simulink model "DynamicCenterGravity_TestModel"  (R2014a)
settings: Solver=ode45  StartTime=0.0  StopTime=10.0  RelTol=1e-3
libraries: rocket_dynamic_data_library x1
settings Model: Creator=scorpii  LastModifiedBy=scorpii

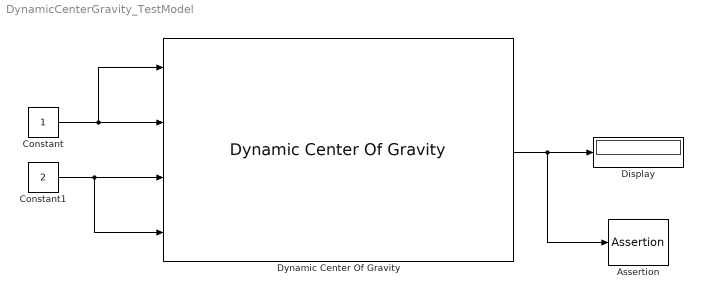
== system DynamicCenterGravity_TestModel ==
  Assertion : Assertion
  Constant : Constant
  Constant1 : Constant  Value=2
  Display : Display
  Dynamic Center Of Gravity : rocket_dynamic_data_library/Dynamic Center Of Gravity
  wires:
  Dynamic Center Of Gravity/1 -> Assertion/1, Display/1
  Constant/1 -> Dynamic Center Of Gravity/1, Dynamic Center Of Gravity/2
  Constant1/1 -> Dynamic Center Of Gravity/4, Dynamic Center Of Gravity/3
